simulink library "DiSC_ToolboxOpal_V12"  (R2012b)
settings: Solver=ode45  StartTime=0.0  StopTime=10.0  RelTol=1e-3
undefined symbols (not defined in the file or in its folder): SamplingTime
(part 5 of 5)

== matlab function DiSC_ToolboxOpal_V12/WindPowerPlant/wtAssetDO5/MATLAB Function ==
  data: p output; wind input; vMeas input; dP input; dPlim input; qRef input; qMode input; vRef input; time input; q output; pAva output
function [p,q,pAva] = wtAssetSDO(wind,vMeas,dP,dPlim,qRef,qMode,vRef, time)
%#codegen
    %wtAssetS implements a simple P,Q controllable wind turbine system for Simulink.
    % This model works for Simulink and requires generatedWindFiles to
    % have been executed before running the simulink model
    % 
    %   The wtAsset can be set to follow an active power reference, output
    %   maximum power available or curtail power. It can also, at the same
    %   time be set to follow a reactive power reference, output the
    %   minimum reactive power according to the power factor or try to keep
    %   a voltage reference in the coupling point by controlling reactive
    %   power output.
    %   
    %   The model is partly based on the book
    %   "Optimal Control of Wind Energy Systems 2008".
    %   
    %   
    % Revision:
    % 23-05-2014, C. E. Sloth and R. Pedersen, Aalborg University. Notes:
    % 29-11-2014, R. Olsen/M. Kemal, Aalborg University (Simulink)
         %Parameters
        param.vBase = 20e3;               % Voltage base [V].
        param.pRated = 100e3;               % Rated output power [W].
        param.sMax = 100e3;                 % Maximum apparent power [VA].
        param.wMin = 3;                   % Cut-in wind speed [m/s].
        param.wMax = 25;                  % Cut-out wind speed [m/s].
        param.wRated = 12;                % Rated wind speed [m/s].
        param.rfTau = 20;                 % Time constant of rotor filter [s].
        param.PF = 1;                     % Power factor [-].
        param.Ts = 60;                    % Sampling time [sec].  

     %variables 
     persistent var;
     if isempty(var)         
        var.p_c=0;                      %All used for caching in between sampling period
        var.q_c=0;
        var.pAva_c=0;
        var.t_c=0;
        var.pOld = 0;                   % [w]. Place holder for the rotor initia filter
        
        var.avgFilterTime = 10*60;      % [s]. Time that the filter should look back 
        var.avgFilterBuf = zeros(ceil(10*60/60),1);
        var.Qmode = 0;                  % [-]. Reactive power control mode
        var.kWT = 3e6/(12^3);           % [-]. Gain from w^3 to p
     end

            % Power conversion constant
            var.kWT = param.pRated/(param.wRated^3);    
            
            % Implement algorithm. 
            
            if (param.Ts>0)
               if (time>(var.t_c+param.Ts))
                   [p,q,pAva,varNew] = sampleWT(param,var,wind,vMeas,dP,dPlim,qRef,vRef);
                   varNew.p_c=p;
                   varNew.q_c=q;
                   varNew.pAva_c=pAva;
                   varNew.t_c=time;
                   varNew.Qmode = qMode;
                   var=varNew;
               end
               p=var.p_c;
               q=var.q_c;
               pAva=var.pAva_c;
            else
                [p,q,pAva,varNew] = sampleWT(param,var,wind,vMeas,dP,dPlim,qRef,vRef);
                var=varNew;
            end
            
        
            
%          [p,q,pAva,varNew] = sampleWT(obj,var,wind,vMeas,dP,dPlim,qRef,vRef);
         
         
end
